simulink model "lookup_nD_TestGen31"  (R2017b)
settings: Solver=FixedStepDiscrete  StartTime=0.0  StopTime=10.0  RelTol=1e-3
settings Model: Creator=ktrinh  LastModifiedBy=ktrinh
settings DebuggingCC: ParameterOverflowMsg=none

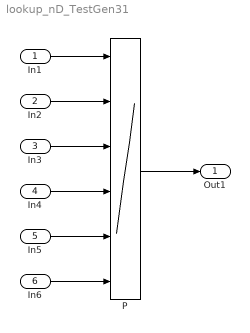
== system lookup_nD_TestGen31 ==
  In1 : Inport  OutMin=0  OutMax=127  OutDataTypeStr=single  PortDimensions=1
  In2 : Inport  Port=2  OutMin=0  OutMax=127  OutDataTypeStr=single
  In3 : Inport  Port=3  OutMin=0  OutMax=127  OutDataTypeStr=single
  In4 : Inport  Port=4  OutMin=0  OutMax=127  OutDataTypeStr=single
  In5 : Inport  Port=5  OutMin=0  OutMax=127  OutDataTypeStr=single
  In6 : Inport  Port=6  OutMin=0  OutMax=127  OutDataTypeStr=single
  P : Lookup_n-D  NumberOfTableDimensions=6  BreakpointsForDimension1=[11.85469112803;64.874153220493]  BreakpointsForDimension2=[2.95942596612804;10.8586691122755;51.2896084520372;86.6441080283528;94.9346929416005]  BreakpointsForDimension3=[14.8298960066499;83.4295978319009;95.7432268121904]  BreakpointsForDimension4=[15.2489263217398;89.3720211330674]  BreakpointsForDimension5=[18.109237470221;32.9710200874685;87.1106088723667]  BreakpointsForDimension6=[12.1492307344412;48.7080133378592;56.5392845021987;102.624951287744]  BreakpointsForDimension1DataTypeStr=int16  BreakpointsForDimension2DataTypeStr=int16  BreakpointsForDimension3DataTypeStr=int16  BreakpointsForDimension4DataTypeStr=int16  BreakpointsForDimension5DataTypeStr=int16  BreakpointsForDimension6DataTypeStr=int16  Table=reshape(repmat([4 5 6 7 8;16 19 20 21 22;10 18 23 24 25],6,8),[2,5,3,2,3, 4])  TableDataTypeStr=double  InterpMethod=Flat  ExtrapMethod=Clip  UseLastTableValue=on  InternalRulePriority=Speed  OutDataTypeStr=Inherit: Inherit from 'Table data'  RndMeth=Nearest  SaturateOnIntegerOverflow=on  InputSameDT=on
  Out1 : Outport
  wires:
  In1/1 -> P/1
  In2/1 -> P/2
  In3/1 -> P/3
  In4/1 -> P/4
  In5/1 -> P/5
  In6/1 -> P/6
  P/1 -> Out1/1
